simulink model "rtwdemo_graphical"  (Simulink 7.1)
settings: Solver=FixedStepDiscrete  StartTime=0.0  StopTime=10.0  RelTol=1e-3
settings Model: Creator=ajayaram  LastModifiedBy=ajayaram
settings OptimizationCC: InlineParams=on  OptimizeModelRefInitCode=on  LifeSpan=1
settings RTWCC: SystemTargetFile=ert.tlc  GenCodeOnly=on  GenerateMakefile=off  TemplateMakefile=ert_default_tmf  Description=Real-Time Workshop Embedded Coder (no auto configuration)  GenerateReport=on  ProcessScript=ert_make_rtw_hook  IncludeHyperlinkInReport=on  LaunchReport=on
settings CodeAppCC: IgnoreCustomStorageClasses=off
settings ERTTargetCC: GenerateSampleERTMain=on  InlinedParameterPlacement=NonHierarchical  ERTCustomFileTemplate=example_file_process.tlc

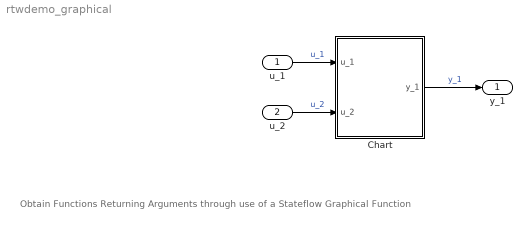
== system rtwdemo_graphical ==
  note: Obtain Functions Returning Arguments
      | through use of a Stateflow Graphical Function
  u_1 : Inport  OutDataType=sfix(16)  OutScaling=2^0
  u_2 : Inport  Port=2  OutDataType=sfix(16)  OutScaling=2^0
  Chart : Stateflow chart
  y_1 : Outport  OutDataType=sfix(16)  OutScaling=2^0
  wires:
  u_1/1 -> Chart/1(u_1)  "u_1"
  Chart/1(y_1) -> y_1/1  "y_1"
  u_2/1 -> Chart/2(u_2)  "u_2"

== stateflow chart Chart ==
  state output = adder(in1, in2) [function]
    (default) -> (junction 6)
    (junction 6) -> (junction 7) : {
        |   output = in1 + in2 ;
        | }
  (junction 4) -> (junction 5) : {
      | y_1 = adder(u_1,u_2);
      | }
  (default) -> (junction 4)
  data: in1 function_input double; in2 function_input double; output function_output double; u_1 input double; u_2 input double; y_1 output double
